simulink model "tcc"  (R2017a)
settings: Solver=ode45  StartTime=0.0  StopTime=10.0  RelTol=1e-3
settings Model: Creator=arthurmoriggipimenta  LastModifiedBy=arthurmoriggipimenta

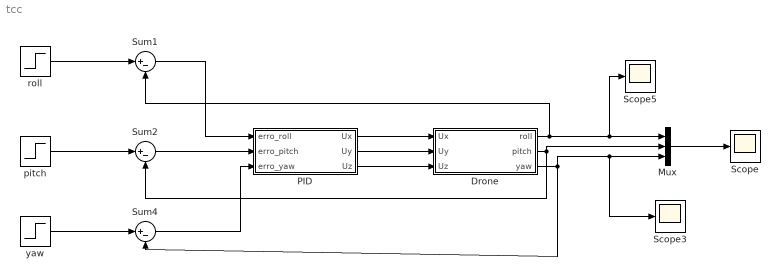
== system tcc ==
  Drone : Subsystem
  Mux : Mux  Inputs=3
  PID : Subsystem
  Scope : Scope
  Scope3 : Scope
  Scope5 : Scope
  Sum1 : Sum  Inputs=|+-
  Sum2 : Sum  Inputs=|+-
  Sum4 : Sum  Inputs=|+-
  pitch : Step  Time=0  After=3.1413/6  SampleTime=0
  roll : Step  Time=0  After=30  SampleTime=30
  yaw : Step  Time=0  After=3.1413/6  SampleTime=0
  wires:
  Drone/2(pitch) -> Sum2/2, Mux/2
  pitch/1 -> Sum2/1
  Drone/3(yaw) -> Sum4/2, Scope3/1, Mux/3
  Drone/1(roll) -> Sum1/2, Scope5/1, Mux/1
  Sum1/1 -> PID/1(erro_roll)
  Sum2/1 -> PID/2(erro_pitch)
  yaw/1 -> Sum4/1
  roll/1 -> Sum1/1
  Sum4/1 -> PID/3(erro_yaw)
  Mux/1 -> Scope/1
  PID/1(Ux) -> Drone/1(Ux)
  PID/3(Uz) -> Drone/3(Uz)
  PID/2("Uy ") -> Drone/2(Uy)

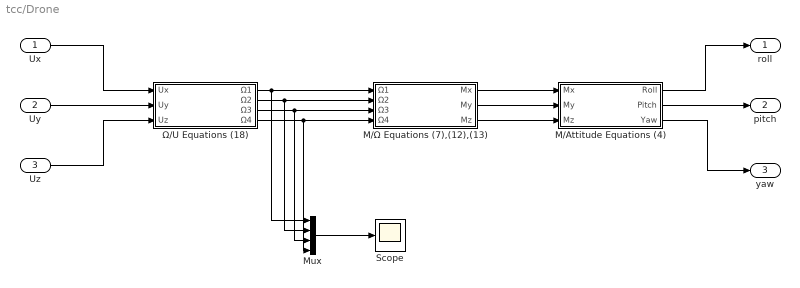
== system tcc/Drone ==
  Ux : Inport
  Uy : Inport  Port=2
  Uz : Inport  Port=3
  " M/Attitude Equations (4)" : Subsystem
  " M/Ω Equations (7),(12),(13)" : Subsystem
  " Ω/U Equations (18)" : Subsystem
  Mux : Mux
  Scope : Scope
  roll : Outport
  pitch : Outport  Port=2
  yaw : Outport  Port=3
  wires:
  Ux/1 -> " Ω/U Equations (18)"/1(Ux)
  Uy/1 -> " Ω/U Equations (18)"/2(Uy)
  Uz/1 -> " Ω/U Equations (18)"/3(Uz)
  " Ω/U Equations (18)"/1(Ω1) -> Mux/1, " M/Ω Equations (7),(12),(13)"/1(Ω1)
  " Ω/U Equations (18)"/3(Ω3) -> Mux/3, " M/Ω Equations (7),(12),(13)"/3(Ω3)
  " Ω/U Equations (18)"/4(Ω4) -> Mux/4, " M/Ω Equations (7),(12),(13)"/4(Ω4)
  " M/Attitude Equations (4)"/2(Pitch) -> pitch/1
  " M/Ω Equations (7),(12),(13)"/1(Mx) -> " M/Attitude Equations (4)"/1(Mx)
  " M/Ω Equations (7),(12),(13)"/2(My) -> " M/Attitude Equations (4)"/2(My)
  " M/Ω Equations (7),(12),(13)"/3(Mz) -> " M/Attitude Equations (4)"/3(Mz)
  " M/Attitude Equations (4)"/1(Roll) -> roll/1
  " M/Attitude Equations (4)"/3(Yaw) -> yaw/1
  " Ω/U Equations (18)"/2(Ω2) -> Mux/2, " M/Ω Equations (7),(12),(13)"/2(Ω2)
  Mux/1 -> Scope/1

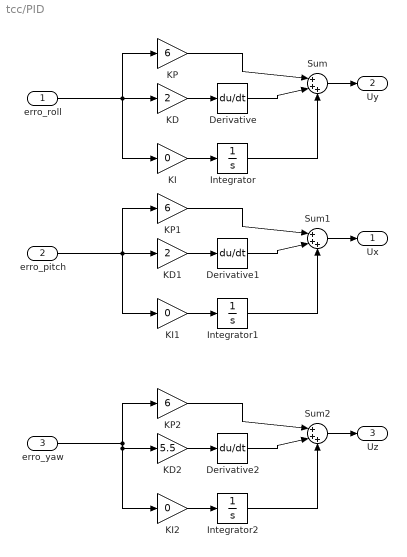
== system tcc/PID ==
  erro_roll : Inport
  erro_pitch : Inport  Port=2
  erro_yaw : Inport  Port=3
  Derivative : Derivative
  Derivative1 : Derivative
  Derivative2 : Derivative
  Integrator : Integrator
  Integrator1 : Integrator
  Integrator2 : Integrator
  KD : Gain  Gain=2
  KD1 : Gain  Gain=2
  KD2 : Gain  Gain=5.5
  KI : Gain  Gain=0
  KI1 : Gain  Gain=0
  KI2 : Gain  Gain=0
  KP : Gain  Gain=6
  KP1 : Gain  Gain=6
  KP2 : Gain  Gain=6
  Sum : Sum  Inputs=|+++
  Sum1 : Sum  Inputs=|+++
  Sum2 : Sum  Inputs=|+++
  Ux : Outport
  "Uy " : Outport  Port=2
  Uz : Outport  Port=3
  wires:
  Sum/1 -> "Uy "/1
  KI/1 -> Integrator/1
  erro_roll/1 -> KI/1, KD/1, KP/1
  KP/1 -> Sum/1
  Derivative/1 -> Sum/2
  Integrator/1 -> Sum/3
  KD/1 -> Derivative/1
  Sum1/1 -> Ux/1
  KI1/1 -> Integrator1/1
  erro_pitch/1 -> KP1/1, KI1/1, KD1/1
  KP1/1 -> Sum1/1
  Derivative1/1 -> Sum1/2
  Integrator1/1 -> Sum1/3
  KD1/1 -> Derivative1/1
  Sum2/1 -> Uz/1
  KI2/1 -> Integrator2/1
  erro_yaw/1 -> KI2/1, KD2/1, KP2/1
  KP2/1 -> Sum2/1
  Derivative2/1 -> Sum2/2
  Integrator2/1 -> Sum2/3
  KD2/1 -> Derivative2/1

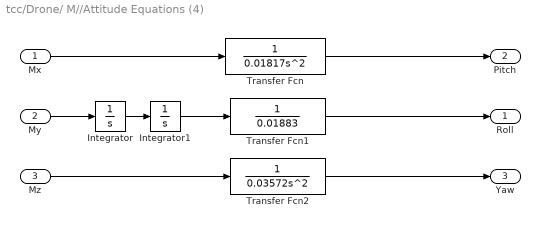
== system tcc/Drone/ M//Attitude Equations (4) ==
  Mx : Inport
  My : Inport  Port=2
  Mz : Inport  Port=3
  Integrator : Integrator
  Integrator1 : Integrator  InitialCondition=3.1413
  Transfer Fcn : TransferFcn  Denominator=[0.01817 0 0]
  Transfer Fcn1 : TransferFcn  Denominator=[0.01883]
  Transfer Fcn2 : TransferFcn  Denominator=[0.03572 0 0]
  Roll : Outport
  Pitch : Outport  Port=2
  Yaw : Outport  Port=3
  wires:
  Transfer Fcn1/1 -> Roll/1
  Transfer Fcn/1 -> Pitch/1
  Transfer Fcn2/1 -> Yaw/1
  Mx/1 -> Transfer Fcn/1
  My/1 -> Integrator/1
  Mz/1 -> Transfer Fcn2/1
  Integrator/1 -> Integrator1/1
  Integrator1/1 -> Transfer Fcn1/1

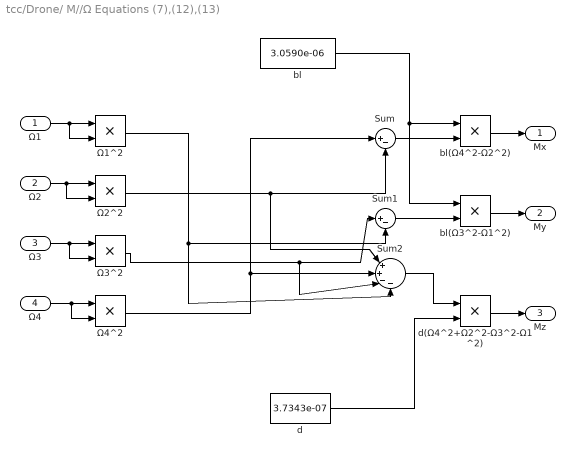
== system tcc/Drone/ M//Ω Equations (7),(12),(13) ==
  Ω1 : Inport
  Ω2 : Inport  Port=2
  Ω3 : Inport  Port=3
  Ω4 : Inport  Port=4
  Sum : Sum  Inputs=|+-
  Sum1 : Sum  Inputs=|+-
  Sum2 : Sum  Inputs=|++--
  bl : Constant  Value=3.0590e-06
  bl(Ω3^2-Ω1^2) : Product
  bl(Ω4^2-Ω2^2) : Product
  d : Constant  Value=3.7343e-07
  d(Ω4^2+Ω2^2-Ω3^2-Ω1^2) : Product
  Ω1^2 : Product
  Ω2^2 : Product
  Ω3^2 : Product
  Ω4^2 : Product
  Mx : Outport
  My : Outport  Port=2
  Mz : Outport  Port=3
  wires:
  Ω1/1 -> Ω1^2/2, Ω1^2/1
  Ω4/1 -> Ω4^2/2, Ω4^2/1
  Ω3/1 -> Ω3^2/2, Ω3^2/1
  Ω2/1 -> Ω2^2/2, Ω2^2/1
  bl/1 -> bl(Ω3^2-Ω1^2)/1, bl(Ω4^2-Ω2^2)/1
  Sum/1 -> bl(Ω4^2-Ω2^2)/2
  bl(Ω4^2-Ω2^2)/1 -> Mx/1
  Ω4^2/1 -> Sum2/2, Sum/1
  Ω2^2/1 -> Sum2/1, Sum/2
  d(Ω4^2+Ω2^2-Ω3^2-Ω1^2)/1 -> Mz/1
  bl(Ω3^2-Ω1^2)/1 -> My/1
  Sum1/1 -> bl(Ω3^2-Ω1^2)/2
  Ω3^2/1 -> Sum2/3, Sum1/1
  Ω1^2/1 -> Sum2/4, Sum1/2
  d/1 -> d(Ω4^2+Ω2^2-Ω3^2-Ω1^2)/2
  Sum2/1 -> d(Ω4^2+Ω2^2-Ω3^2-Ω1^2)/1

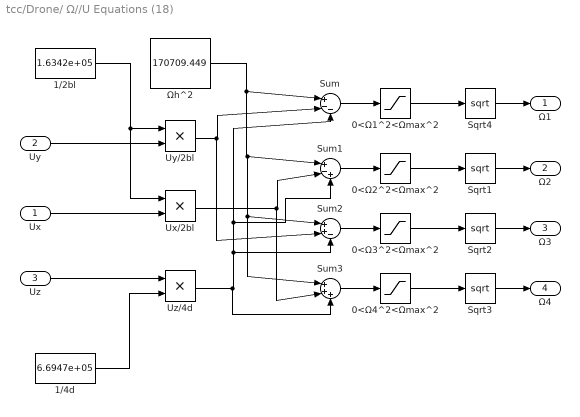
== system tcc/Drone/ Ω//U Equations (18) ==
  Ux : Inport
  Uy : Inport  Port=2
  Uz : Inport  Port=3
  " 0<Ω1^2<Ωmax^2 " : Saturate  UpperLimit=490000  LowerLimit=0  ZeroCross=off
  " 0<Ω2^2<Ωmax^2 " : Saturate  UpperLimit=490000  LowerLimit=0  ZeroCross=off
  " 0<Ω3^2<Ωmax^2 " : Saturate  UpperLimit=490000  LowerLimit=0  ZeroCross=off
  " 0<Ω4^2<Ωmax^2 " : Saturate  UpperLimit=490000  LowerLimit=0  ZeroCross=off
  1/2bl : Constant  Value=1.6342e+05
  1/4d : Constant  Value=6.6947e+05
  Sqrt{1..4} (4 alike) : Sqrt  SaturateOnIntegerOverflow=on
  Sum : Sum  Inputs=|+--
  Sum1 : Sum  Inputs=|+-+
  Sum2 : Sum  Inputs=|++-
  Sum3 : Sum  Inputs=|+++
  Ux/2bl : Product
  Uy/2bl : Product
  Uz/4d : Product
  Ωh^2 : Constant  Value=170709.449
  Ω1 : Outport
  Ω2 : Outport  Port=2
  Ω3 : Outport  Port=3
  Ω4 : Outport  Port=4
  wires:
  Ωh^2/1 -> Sum3/1, Sum2/1, Sum1/1, Sum/1
  Sum/1 -> " 0<Ω1^2<Ωmax^2 "/1
  1/2bl/1 -> Ux/2bl/1, Uy/2bl/1
  Uy/1 -> Uy/2bl/2
  Uy/2bl/1 -> Sum2/2, Sum/2
  1/4d/1 -> Uz/4d/2
  Uz/1 -> Uz/4d/1
  Uz/4d/1 -> Sum3/3, Sum2/3, Sum1/3, Sum/3
  Ux/1 -> Ux/2bl/2
  Sum3/1 -> " 0<Ω4^2<Ωmax^2 "/1
  Sum2/1 -> " 0<Ω3^2<Ωmax^2 "/1
  Sum1/1 -> " 0<Ω2^2<Ωmax^2 "/1
  Ux/2bl/1 -> Sum3/2, Sum1/2
  " 0<Ω1^2<Ωmax^2 "/1 -> Sqrt4/1
  Sqrt4/1 -> Ω1/1
  " 0<Ω4^2<Ωmax^2 "/1 -> Sqrt3/1
  " 0<Ω3^2<Ωmax^2 "/1 -> Sqrt2/1
  " 0<Ω2^2<Ωmax^2 "/1 -> Sqrt1/1
  Sqrt3/1 -> Ω4/1
  Sqrt2/1 -> Ω3/1
  Sqrt1/1 -> Ω2/1
